simulink model "prototype_for_iterator_from_zero"  (R2021b)
settings: Solver=FixedStepAuto  StartTime=0.0  StopTime=10.0  FixedStep=1  RelTol=1e-3
settings Model: Creator=grodriguez  LastModifiedBy=grodriguez
settings OptimizationCC: DefaultParameterBehavior=Inlined  EnhancedBackFolding=on  PassReuseOutputArgsAs=Individual arguments  ZeroExternalMemoryAtStartup=off  ZeroInternalMemoryAtStartup=off  OptimizeBlockOrder=speed  DifferentSizesBufferReuse=on  OptimizationCustomize=off  EfficientTunableParamExpr=on
settings DebuggingCC: ParameterTunabilityLossMsg=error
settings SFSimCC: MATLABDynamicMemAlloc=off
settings RTWCC: Description=Embedded Coder  SystemTargetFile=ert.tlc  GenCodeOnly=on  TemplateMakefile=ert_default_tmf
settings CodeAppCC: ForceParamTrailComments=on  IgnoreCustomStorageClasses=off  OperatorAnnotations=on  SimulinkDataObjDesc=on  SFDataObjDesc=on  InsertBlockDesc=on
settings ERTTargetCC: TargetLangStandard=C99 (ISO)  GenerateSampleERTMain=on  InlinedParameterPlacement=NonHierarchical  ERTCustomFileTemplate=example_file_process.tlc

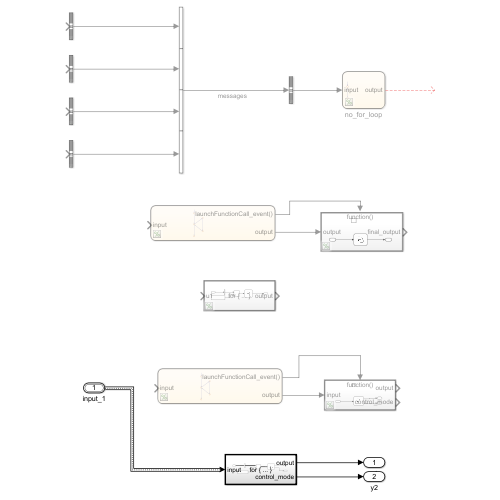
[thumbnail: Simulink's stored preview of the top-level diagram]
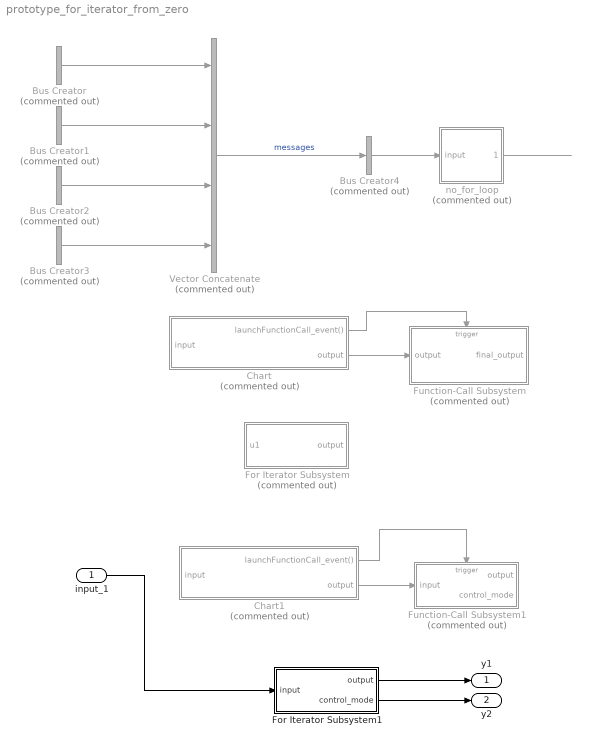
== system prototype_for_iterator_from_zero ==
  input_1 : Inport  OutDataTypeStr=Bus: BUS_MESSAGES_RX_MULTIPLE  BusOutputAsStruct=on
  Bus Creator{,1..3} (4 alike) : BusCreator  Commented=on  Inputs=1  OutDataTypeStr=Bus: BUS_MESSAGES_RX  NonVirtualBus=on
  Bus Creator4 : BusCreator  Commented=on  Inputs=1  OutDataTypeStr=Bus: BUS_MESSAGES_RX_MULTIPLE
  Chart : Stateflow chart  Commented=on  TreatAsAtomicUnit=on
      settings: PortSchema="{\"entries\":[{\"content\":{\"sides\":[{\"content\":{\"connectorIds\":[\"In1\"]},\"type\":\"ConnectorPlacement.EquallySpacedRectSide\",\"uuid\":\"25437ac9-0672-44d5-b5ae-7fac701ea7b6\"},{\"content\":{\"connectorIds\":[\"Out2\",\"Out1\"],\"side\":\"RIGHT\"},\"type\":\"ConnectorPlacement.EquallySpacedRectSide\",\"uuid\":\"d00bbbd5-2497-4a00-aca0-7696dceb38fb\"},{\"content\":{\"connectorIds\":[],\"side\":\"TOP\"},\"type\":\"ConnectorPlacement.EquallySpacedRectSide\",\"uuid\":\"e3fbf99c-7202-46f5-80be-3c9f45bd91c9\"}]},\"type\":\"ConnectorPlacement.EquallySpacedConnector\",\"uuid\":\"5faa8b09-f7f1-4bbd-9b0a-4f86c0c2feb9\"}],\"packageUris\":[\"http://schema.mathworks.com/mf0/Connector/R2020b\"],\"version\":\"1.0\"}"
  Chart1 : Stateflow chart  Commented=on  TreatAsAtomicUnit=on
      settings: PortSchema="{\"entries\":[{\"content\":{\"sides\":[{\"content\":{\"connectorIds\":[\"In1\"]},\"type\":\"ConnectorPlacement.EquallySpacedRectSide\",\"uuid\":\"25437ac9-0672-44d5-b5ae-7fac701ea7b6\"},{\"content\":{\"connectorIds\":[\"Out2\",\"Out1\"],\"side\":\"RIGHT\"},\"type\":\"ConnectorPlacement.EquallySpacedRectSide\",\"uuid\":\"d00bbbd5-2497-4a00-aca0-7696dceb38fb\"},{\"content\":{\"connectorIds\":[],\"side\":\"TOP\"},\"type\":\"ConnectorPlacement.EquallySpacedRectSide\",\"uuid\":\"e3fbf99c-7202-46f5-80be-3c9f45bd91c9\"}]},\"type\":\"ConnectorPlacement.EquallySpacedConnector\",\"uuid\":\"5faa8b09-f7f1-4bbd-9b0a-4f86c0c2feb9\"}],\"packageUris\":[\"http://schema.mathworks.com/mf0/Connector/R2020b\"],\"version\":\"1.0\"}"
  For Iterator Subsystem : Subsystem  Commented=on  TreatAsAtomicUnit=on
  For Iterator Subsystem1 : Subsystem  TreatAsAtomicUnit=on
  Function-Call Subsystem : Subsystem  Commented=on  TreatAsAtomicUnit=on
  Function-Call Subsystem1 : Subsystem  Commented=on  TreatAsAtomicUnit=on
  Vector Concatenate : Concatenate  Commented=on  NumInputs=4
  no_for_loop : Stateflow chart  Commented=on  TreatAsAtomicUnit=on
  y1 : Outport  OutDataTypeStr=double
  y2 : Outport  Port=2  OutDataTypeStr=int32
  wires:
  Bus Creator3/1 -> Vector Concatenate/4
  Bus Creator2/1 -> Vector Concatenate/3
  Bus Creator1/1 -> Vector Concatenate/2
  Bus Creator/1 -> Vector Concatenate/1
  Vector Concatenate/1 -> Bus Creator4/1  "messages"
  Bus Creator4/1 -> no_for_loop/1(input)
  no_for_loop/1(output) -> ?
  Chart/1(output) -> Function-Call Subsystem/1(output)
  Chart/2(launchFunctionCall_event()) -> Function-Call Subsystem/Trigger
  Chart1/1(output) -> Function-Call Subsystem1/1(input)
  Chart1/2(launchFunctionCall_event()) -> Function-Call Subsystem1/Trigger
  For Iterator Subsystem1/1(output) -> y1/1
  For Iterator Subsystem1/2(control_mode) -> y2/1
  input_1/1 -> For Iterator Subsystem1/1(input)

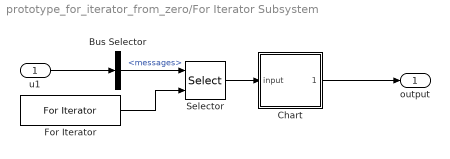
== system prototype_for_iterator_from_zero/For Iterator Subsystem ==
  u1 : Inport  OutDataTypeStr=Bus: BUS_MESSAGES_RX_MULTIPLE
  Bus Selector : BusSelector  OutputSignals=messages
  Chart : Stateflow chart  TreatAsAtomicUnit=on
  For Iterator : ForIterator
  Selector : Selector  NumberOfDimensions=2  InputPortWidth=3  IndexOptions=Index vector (dialog),Index vector (port)  Indices=1,1  OutputSizes=1,1
  output : Outport  OutDataTypeStr=int32
  wires:
  u1/1 -> Bus Selector/1
  Bus Selector/1 -> Selector/1  "<messages>"
  For Iterator/1 -> Selector/2
  Selector/1 -> Chart/1(input)
  Chart/1(output) -> output/1

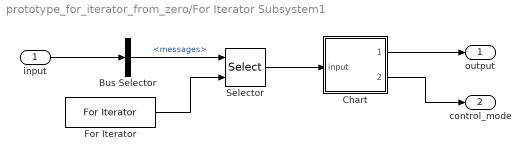
== system prototype_for_iterator_from_zero/For Iterator Subsystem1 ==
  input : Inport  OutDataTypeStr=Bus: BUS_MESSAGES_RX_MULTIPLE
  Bus Selector : BusSelector  OutputSignals=messages
  Chart : Stateflow chart  TreatAsAtomicUnit=on
  For Iterator : ForIterator  IterationLimit=4
  Selector : Selector  NumberOfDimensions=2  InputPortWidth=3  IndexOptions=Index vector (dialog),Index vector (port)  Indices=1,1  OutputSizes=1,1
  output : Outport  OutDataTypeStr=double
  control_mode : Outport  Port=2  OutDataTypeStr=int32
  wires:
  For Iterator/1 -> Selector/2
  Selector/1 -> Chart/1(input)
  Chart/1(output) -> output/1
  Chart/2(control_mode) -> control_mode/1
  input/1 -> Bus Selector/1
  Bus Selector/1 -> Selector/1  "<messages>"

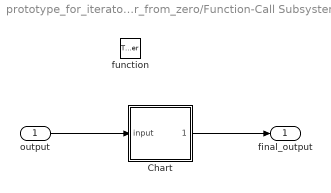
== system prototype_for_iterator_from_zero/Function-Call Subsystem ==
  output : Inport  OutDataTypeStr=Bus: BUS_MESSAGES_RX
  function : TriggerPort  TriggerType=function-call  VariantControl=(inherit)
  Chart : Stateflow chart  TreatAsAtomicUnit=on
  final_output : Outport  OutDataTypeStr=int32
  wires:
  output/1 -> Chart/1(input)
  Chart/1(output) -> final_output/1

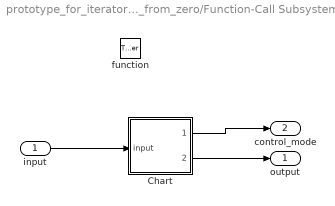
== system prototype_for_iterator_from_zero/Function-Call Subsystem1 ==
  input : Inport  OutDataTypeStr=Bus: BUS_MESSAGES_RX
  function : TriggerPort  TriggerType=function-call  VariantControl=(inherit)
  Chart : Stateflow chart  TreatAsAtomicUnit=on
  output : Outport  OutDataTypeStr=double
  control_mode : Outport  Port=2  OutDataTypeStr=int32
  wires:
  input/1 -> Chart/1(input)
  Chart/2(output) -> output/1
  Chart/1(control_mode) -> control_mode/1

== stateflow chart prototype_for_iterator_from_zero/Chart ==
  (default) -> (junction 5)
  (junction 5) -> (junction 7) : {index = 1;}
  (junction 7) -> (junction 9) [order 1] : [index <= 4]
  (junction 9) -> (junction 11) : {output = input.messages(index); send(launchFunctionCall_event)}
  (junction 11) -> (junction 7) : {index = index + 1;}
  (junction 7) -> (junction 14) [order 2]
  data: index local double size=1 =1; input input Bus: BUS_MESSAGES_RX_MULTIPLE size=1; output output Bus: BUS_MESSAGES_RX size=1
  events: launchFunctionCall_event output FUNCTION_CALL_EVENT

== stateflow chart prototype_for_iterator_from_zero/Function-Call Subsystem/Chart ==
  state init
  (default) -> init
  (junction 10) -> init
  init -> (junction 10) : {output = output + input.control_mode;}
  data: input input Bus: BUS_MESSAGES_RX; output output int32 =int32(0)

== stateflow chart prototype_for_iterator_from_zero/no_for_loop ==
  (default) -> (junction 1)
  (junction 1) -> (junction 5) : {output = input.messages(3).control_mode;}
  data: output output int32; input input Bus: BUS_MESSAGES_RX_MULTIPLE

== stateflow chart prototype_for_iterator_from_zero/For Iterator Subsystem/Chart ==
  state init
  (default) -> init
  (junction 4) -> init
  init -> (junction 4) : {output = output + input.control_mode;}
  data: input input Bus: BUS_MESSAGES_RX; output output int32 =int32(0)

== stateflow chart prototype_for_iterator_from_zero/Chart1 ==
  (default) -> (junction 5)
  (junction 5) -> (junction 7) : {index = 1;}
  (junction 7) -> (junction 9) [order 1] : [index <= 4]
  (junction 9) -> (junction 11) : {output = input.messages(index); send(launchFunctionCall_event)}
  (junction 11) -> (junction 7) : {index = index + 1;}
  (junction 7) -> (junction 14) [order 2]
  data: index local double size=1 =1; input input Bus: BUS_MESSAGES_RX_MULTIPLE size=1; output output Bus: BUS_MESSAGES_RX size=1
  events: launchFunctionCall_event output FUNCTION_CALL_EVENT

== stateflow chart prototype_for_iterator_from_zero/Function-Call Subsystem1/Chart ==
  state idle
    entry:
    control_mode = input.control_mode;
    output = 100;
  state running
    entry:
    control_mode = input.control_mode;
    output = 200;
  state fault
    entry:
    control_mode = input.control_mode;
    output = 300;
  (default) -> idle
  idle -> running : [input.control_mode == 1]
  fault -> idle : [input.control_mode == 0]
  running -> fault : [input.control_mode == -1]
  data: input input Bus: BUS_MESSAGES_RX; control_mode output int32; output output double

== stateflow chart prototype_for_iterator_from_zero/For Iterator Subsystem1/Chart ==
  state init
    entry:
    control_mode = input.control_mode
    output = 100;
  state running
    entry:
    control_mode = input.control_mode
    output = 200;
  state fault
    entry:
    control_mode = input.control_mode
    output = 300;
  (default) -> init
  init -> running : [input.control_mode == 1]
  fault -> init : [input.control_mode == 0]
  running -> fault : [input.control_mode == -1]
  data: input input Bus: BUS_MESSAGES_RX; output output double; control_mode output int32
